simulink model "helicopter"  (R2017a)
settings: Solver=ode45  StartTime=0.0  StopTime=30  RelTol=1e-3  EnableMultiTasking=on
model workspace (MAT data in the model file):
  Con = 0
  Gai = 0
values from neighbouring files (symbols this model uses):
  i = i-1    (= 0)    [expand_subsystem.m]
undefined symbols (not defined in the file or in its folder): a
settings Model: Creator=alex  LastModifiedBy=nikhil
settings DataIOCC: LimitDataPoints=on  SaveFormat=Array
settings OptimizationCC: LifeSpan=inf
settings DebuggingCC: SFUnexpectedBacktrackingDiag=warning  SFNoUnconditionalDefaultTransitionDiag=warning  SFExecutionAtInitializationDiag=none
settings HardwareCC: ProdBitPerPointer=32  ProdBitPerSizeT=32  ProdBitPerPtrDiffT=32  ProdLargestAtomicFloat=None  ProdIntDivRoundTo=Undefined  ProdEndianess=Unspecified  ProdWordSize=32  ProdHWDeviceType=32-bit Generic
settings ModelReferenceCC: PropagateSignalLabelsOutOfModel=off
settings GRTTargetCC: TargetLangStandard=C89/C90 (ANSI)  GeneratePreprocessorConditionals=Disable all
settings ConfigComp: CovMetricSettings=dw  CovHtmlReporting=on  CovSaveCumulativeToWorkspaceVar=on  CovSaveSingleToWorkspaceVar=on  CovExternalEMLEnable=off  CovSFcnEnable=off

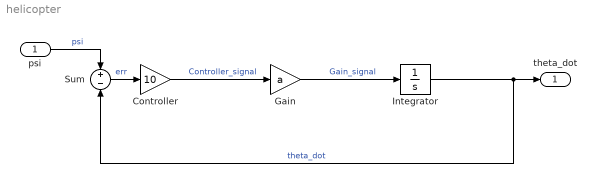
== system helicopter ==
  psi : Inport
  Controller : Gain  Gain=10
  Gain : Gain  Gain=a
  Integrator : Integrator  InitialCondition=i
  Sum : Sum  Inputs=+-
  theta_dot : Outport
  wires:
  Gain/1 -> Integrator/1  "Gain_signal"
  Integrator/1 -> Sum/2, theta_dot/1  "theta_dot"
  Controller/1 -> Gain/1  "Controller_signal"
  psi/1 -> Sum/1  "psi"
  Sum/1 -> Controller/1  "err"
